simulink model "sistem_ordin_I_cu_timp_mort_cu_integrator"  (R2023b)
settings: Solver=VariableStepAuto  StartTime=0.0  StopTime=100  MaxStep=1e-3  RelTol=1e-3
values from neighbouring files (symbols this model uses):
  b = 0.2    [sns_proiect_Ceoca_Ovidiu.m]
  den = [T 1]    [sns_proiect_Ceoca_Ovidiu.m]
  h1 = T/10    (= 0.2)    [sns_proiect_Ceoca_Ovidiu.m]
  Kp = 0.45*Ku    (= 0.450881601519)    [sns_proiect_Ceoca_Ovidiu.m]
  num = [1]    [sns_proiect_Ceoca_Ovidiu.m]
  taum = 1    [sns_proiect_Ceoca_Ovidiu.m]
  Ti = 0.8*Tosc    (= 8)    [sns_proiect_Ceoca_Ovidiu.m]
  Tt1 = 0.5    [sns_proiect_Ceoca_Ovidiu.m]
settings Model: Creator=ovidiuceoca  LastModifiedBy=ovidiuceoca

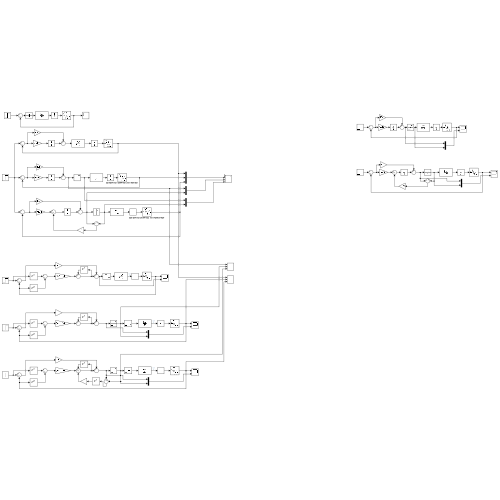
[thumbnail: Simulink's stored preview of the top-level diagram]
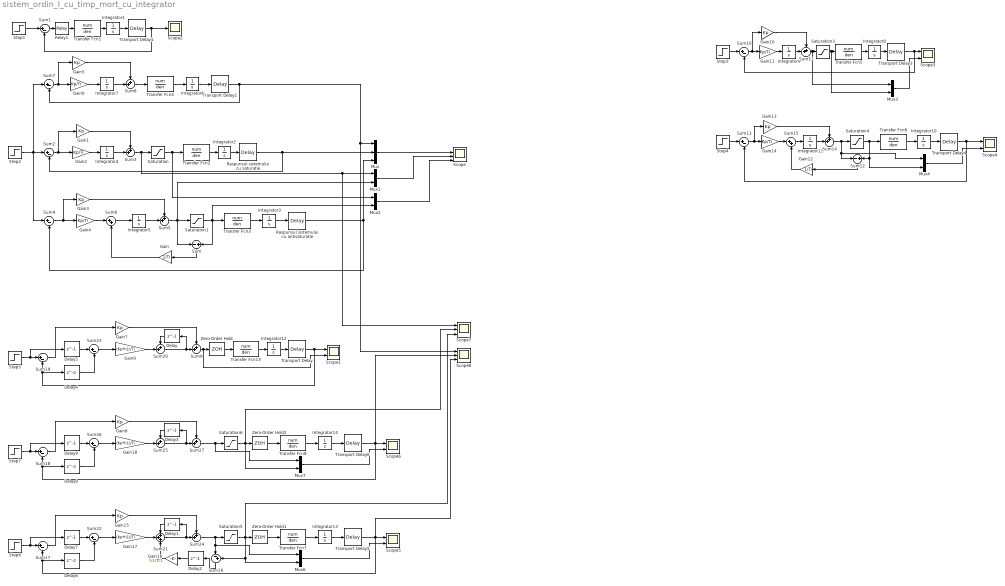
== system sistem_ordin_I_cu_timp_mort_cu_integrator ==
  Delay{,1..3,5,7,9} (7 alike) : Delay  DelayLength=1  SampleTime=h1
  Delay4 : Delay  SampleTime=h1
  Delay6 : Delay  SampleTime=h1
  Delay8 : Delay  SampleTime=h1
  Gain : Gain  Gain=1/Ti
  Gain{1,3,5,7..8,10,13,15} (8 alike) : Gain  Gain=Kp
  Gain{2,4,6,11,14} (5 alike) : Gain  Gain=Kp/Ti
  Gain12 : Gain  Gain=1/Ti
  Gain16 : Gain  Gain=h1/Tt1
  Gain17 : Gain  Gain=(Kp*h1)/Ti
  Gain18 : Gain  Gain=(Kp*h1)/Ti
  Gain9 : Gain  Gain=(Kp*h1)/Ti
  Integrator{1..14} (14 alike) : Integrator
  Mux : Mux  Inputs=3
  Mux{1..4,6..7} (6 alike) : Mux  Inputs=2
  Raspunsul sistemului cu antisaturatie : TransportDelay  DelayTime=taum
  Raspunsul sistemului cu saturatie : TransportDelay  DelayTime=taum
  Relay1 : Relay  OnSwitchValue=0  OffSwitchValue=0  OnOutputValue=b  OffOutputValue=-b
  Saturation : Saturate  UpperLimit=0.2  LowerLimit=-1
  Saturation1 : Saturate  UpperLimit=0.2  LowerLimit=-1
  Saturation3 : Saturate  UpperLimit=0.2  LowerLimit=-0.2
  Saturation4 : Saturate  UpperLimit=0.2  LowerLimit=-0.2
  Saturation5 : Saturate  UpperLimit=0.3  LowerLimit=-0.3
  Saturation6 : Saturate  UpperLimit=0.3  LowerLimit=-0.3
  Scope : Scope  NumInputPorts=4
  Scope{1,3..6} (5 alike) : Scope  NumInputPorts=2
  Scope2 : Scope
  Scope7 : Scope  NumInputPorts=3
  Scope8 : Scope  NumInputPorts=3
  Step1 : Step  Time=0  After=0.5  SampleTime=0
  Step{2..7} (6 alike) : Step  Time=0  SampleTime=0
  Sum : Sum  Inputs=-|+
  Sum{1..2,4,7,10,13,17..19,22..23,26} (12 alike) : Sum  Inputs=|+-
  Sum{3,5,8..9,11,14,20,24..25,27} (10 alike) : Sum  Inputs=++|
  Sum12 : Sum  Inputs=-|+
  Sum15 : Sum  Inputs=|++
  Sum16 : Sum  Inputs=|-+
  Sum21 : Sum  Inputs=+++
  Sum6 : Sum  Inputs=|++
  Transfer Fcn{1..8,13} (9 alike) : TransferFcn  Numerator=num  Denominator=den
  Transport Delay{,1..6} (7 alike) : TransportDelay  DelayTime=taum
  Zero-Order Hold : ZeroOrderHold  SampleTime=h1
  Zero-Order Hold1 : ZeroOrderHold  SampleTime=h1
  Zero-Order Hold2 : ZeroOrderHold  SampleTime=h1
  wires:
  Step1/1 -> Sum1/1
  Relay1/1 -> Transfer Fcn1/1
  Transfer Fcn1/1 -> Integrator1/1
  Sum1/1 -> Relay1/1
  Integrator1/1 -> Transport Delay1/1
  Saturation/1 -> Mux2/1, Transfer Fcn2/1
  Gain1/1 -> Sum3/1
  Raspunsul sistemului cu saturatie/1 -> Mux/2, Sum2/2
  Integrator4/1 -> Sum3/2
  Gain2/1 -> Integrator4/1
  Integrator2/1 -> Raspunsul sistemului cu saturatie/1
  Transfer Fcn2/1 -> Integrator2/1
  Sum2/1 -> Gain2/1, Gain1/1
  Sum3/1 -> Scope7/1, Mux1/1, Saturation/1
  Transfer Fcn3/1 -> Integrator3/1
  Saturation1/1 -> Mux2/2, Transfer Fcn3/1, Sum/2
  Raspunsul sistemului cu antisaturatie/1 -> Sum4/2, Mux/3
  Sum4/1 -> Gain4/1, Gain3/1
  Gain3/1 -> Sum5/1
  Integrator5/1 -> Sum5/2
  Integrator3/1 -> Raspunsul sistemului cu antisaturatie/1
  Sum5/1 -> Mux1/2, Sum/1, Saturation1/1
  Sum/1 -> Gain/1
  Gain4/1 -> Sum6/1
  Sum6/1 -> Integrator5/1
  Gain/1 -> Sum6/2
  Gain6/1 -> Integrator7/1
  Transfer Fcn4/1 -> Integrator6/1
  Sum8/1 -> Transfer Fcn4/1
  Transport Delay2/1 -> Scope8/1, Mux/1, Sum7/2
  Sum7/1 -> Gain6/1, Gain5/1
  Gain5/1 -> Sum8/1
  Integrator7/1 -> Sum8/2
  Integrator6/1 -> Transport Delay2/1
  Mux/1 -> Scope/2
  Mux1/1 -> Scope/3
  Mux2/1 -> Scope/4
  Sum20/1 -> Sum9/2, Delay/1
  Delay4/1 -> Sum23/2
  Gain9/1 -> Sum20/2
  Zero-Order Hold/1 -> Transfer Fcn13/1
  Delay/1 -> Sum20/1
  Transfer Fcn13/1 -> Integrator12/1
  Sum23/1 -> Gain9/1
  Transport Delay/1 -> Scope1/1, Sum19/2, Delay4/1
  Delay5/1 -> Sum23/1
  Sum19/1 -> Gain7/1
  Gain7/1 -> Sum9/1
  Transport Delay1/1 -> Scope2/1, Sum1/2
  Step2/1 -> Sum7/1, Sum4/1, Sum2/1
  Integrator8/1 -> Transport Delay3/1
  Integrator9/1 -> Sum11/2
  Gain11/1 -> Integrator9/1
  Transport Delay3/1 -> Scope3/1, Sum10/2
  Step3/1 -> Sum10/1
  Gain10/1 -> Sum11/1
  Transfer Fcn5/1 -> Integrator8/1
  Saturation3/1 -> Mux3/2, Transfer Fcn5/1
  Sum11/1 -> Mux3/1, Saturation3/1
  Sum10/1 -> Gain10/1, Gain11/1
  Mux3/1 -> Scope3/2
  Transfer Fcn6/1 -> Integrator10/1
  Sum15/1 -> Integrator11/1
  Transport Delay4/1 -> Scope4/1, Sum13/2
  Gain14/1 -> Sum15/1
  Gain12/1 -> Sum15/2
  Saturation4/1 -> Transfer Fcn6/1, Mux4/2, Sum12/2
  Gain13/1 -> Sum14/1
  Sum14/1 -> Sum12/1, Mux4/1, Saturation4/1
  Integrator10/1 -> Transport Delay4/1
  Sum12/1 -> Gain12/1
  Sum13/1 -> Gain14/1, Gain13/1
  Integrator11/1 -> Sum14/2
  Step4/1 -> Sum13/1
  Mux4/1 -> Scope4/2
  Step5/1 -> Delay5/1, Sum19/1
  Integrator12/1 -> Transport Delay/1
  Sum16/1 -> Delay2/1
  Delay1/1 -> Sum21/1
  Step6/1 -> Delay7/1, Sum17/1
  Transfer Fcn7/1 -> Integrator13/1
  Transport Delay5/1 -> Scope8/3, Scope5/1, Sum17/2, Delay6/1
  Delay2/1 -> Gain16/1
  Sum17/1 -> Gain15/1
  Sum21/1 -> Sum24/2, Delay1/1
  Gain16/1 -> Sum21/3
  Zero-Order Hold1/1 -> Transfer Fcn7/1
  Mux6/1 -> Scope5/2
  Delay6/1 -> Sum22/2
  Gain17/1 -> Sum21/2
  Sum24/1 -> Sum16/1, Mux6/1, Saturation5/1
  Sum22/1 -> Gain17/1
  Integrator13/1 -> Transport Delay5/1
  Delay7/1 -> Sum22/1
  Saturation5/1 -> Scope7/3, Mux6/2, Sum16/2, Zero-Order Hold1/1
  Gain15/1 -> Sum24/1
  Sum18/1 -> Gain8/1
  Delay3/1 -> Sum25/1
  Transport Delay6/1 -> Scope8/2, Scope6/1, Sum18/2, Delay8/1
  Transfer Fcn8/1 -> Integrator14/1
  Step7/1 -> Delay9/1, Sum18/1
  Sum25/1 -> Sum27/2, Delay3/1
  Delay9/1 -> Sum26/1
  Gain18/1 -> Sum25/2
  Mux7/1 -> Scope6/2
  Delay8/1 -> Sum26/2
  Sum27/1 -> Mux7/1, Saturation6/1
  Zero-Order Hold2/1 -> Transfer Fcn8/1
  Sum26/1 -> Gain18/1
  Integrator14/1 -> Transport Delay6/1
  Saturation6/1 -> Scope7/2, Mux7/2, Zero-Order Hold2/1
  Gain8/1 -> Sum27/1
  Sum9/1 -> Scope1/2, Zero-Order Hold/1
